simulink model "p03_PID_ZN_SSA_ISSA"  (R2016a)
settings: Solver=VariableStepAuto  StartTime=0.0  StopTime=100  RelTol=1e-3
libraries: simulink x5, dspsrcs4 x1
settings Model: Creator=Administrator  LastModifiedBy=Administrator

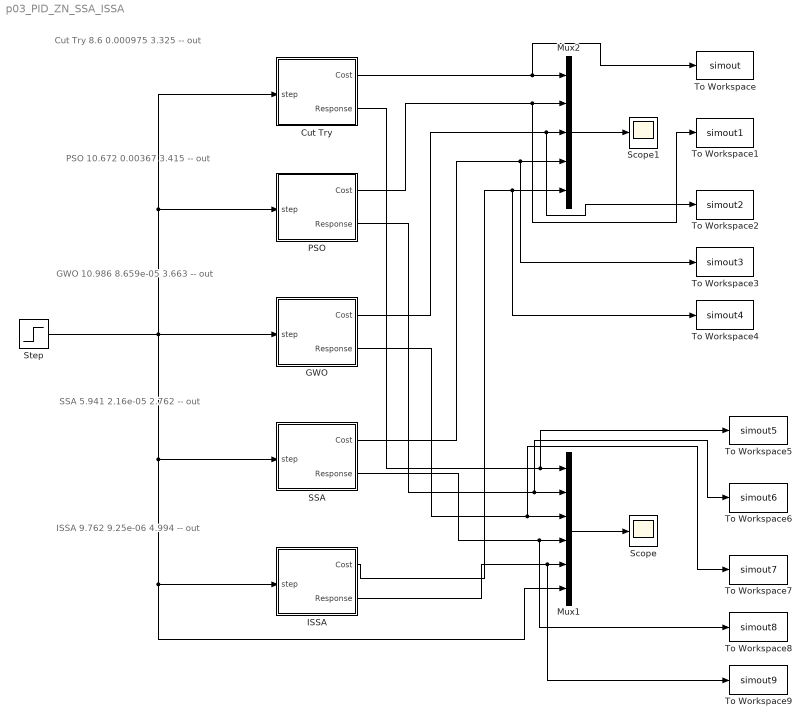
== system p03_PID_ZN_SSA_ISSA ==
  note: ISSA 9.762 9.25e-06 4.994 -- out
  note: SSA 5.941 2.16e-05 2.762 -- out
  note: Cut Try 8.6 0.000975 3.325 -- out
  note: GWO 10.986 8.659e-05 3.663 -- out
  note: PSO 10.672 0.00367 3.415 -- out
  Cut Try : Subsystem
  GWO : Subsystem
  ISSA : Subsystem
  Mux1 : Mux  Inputs=6
  Mux2 : Mux  Inputs=5
  PSO : Subsystem
  SSA : Subsystem
  Scope : Scope
  Scope1 : Scope
  Step : Step  Time=10  SampleTime=0
  To Workspace : ToWorkspace  VariableName=simout  SaveFormat=Timeseries  SampleTime=-1
  To Workspace1 : ToWorkspace  VariableName=simout1  SaveFormat=Timeseries  SampleTime=-1
  To Workspace2 : ToWorkspace  VariableName=simout2  SaveFormat=Timeseries  SampleTime=-1
  To Workspace3 : ToWorkspace  VariableName=simout3  SaveFormat=Timeseries  SampleTime=-1
  To Workspace4 : ToWorkspace  VariableName=simout4  SaveFormat=Timeseries  SampleTime=-1
  To Workspace5 : ToWorkspace  VariableName=simout5  SaveFormat=Timeseries  SampleTime=-1
  To Workspace6 : ToWorkspace  VariableName=simout6  SaveFormat=Timeseries  SampleTime=-1
  To Workspace7 : ToWorkspace  VariableName=simout7  SaveFormat=Timeseries  SampleTime=-1
  To Workspace8 : ToWorkspace  VariableName=simout8  SaveFormat=Timeseries  SampleTime=-1
  To Workspace9 : ToWorkspace  VariableName=simout9  SaveFormat=Timeseries  SampleTime=-1
  wires:
  Mux1/1 -> Scope/1
  Mux2/1 -> Scope1/1
  Step/1 -> GWO/1(step), PSO/1(step), Cut Try/1(step), Mux1/6, ISSA/1(step), SSA/1(step)
  Cut Try/1(Cost) -> To Workspace/1, Mux2/1
  Cut Try/2(Response) -> To Workspace5/1, Mux1/1
  PSO/1(Cost) -> To Workspace1/1, Mux2/2
  PSO/2(Response) -> To Workspace6/1, Mux1/2
  GWO/1(Cost) -> To Workspace2/1, Mux2/3
  GWO/2(Response) -> To Workspace7/1, Mux1/3
  SSA/1(Cost) -> To Workspace3/1, Mux2/4
  SSA/2(Response) -> To Workspace8/1, Mux1/4
  ISSA/1(Cost) -> To Workspace4/1, Mux2/5
  ISSA/2(Response) -> To Workspace9/1, Mux1/5

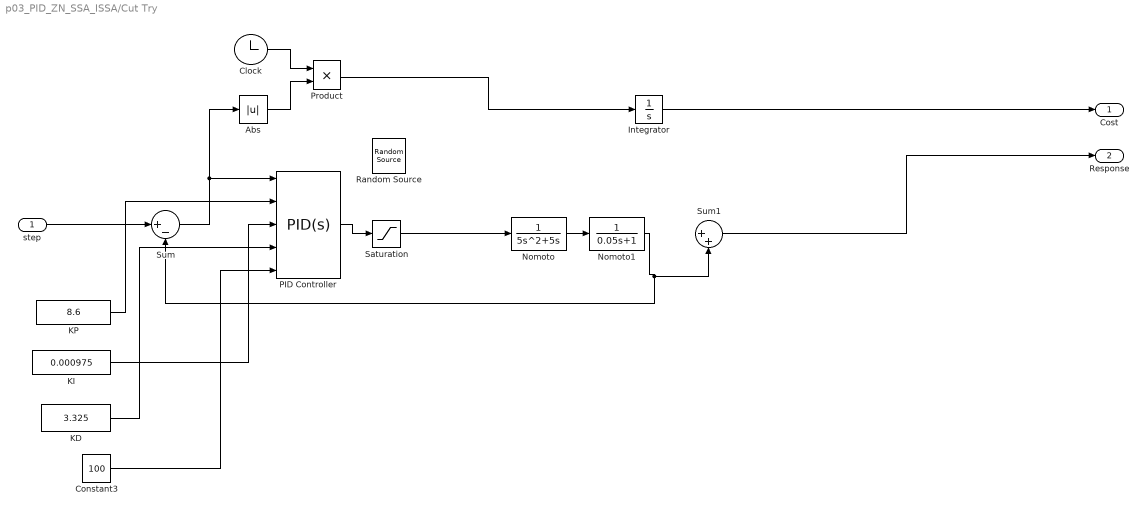
== system p03_PID_ZN_SSA_ISSA/Cut Try ==
  step : Inport
  Abs : Abs
  Clock : Clock
  Constant3 : Constant  Value=100
  Integrator : Integrator
  KD : Constant  Value=3.325
  KI : Constant  Value=0.000975
  KP : Constant  Value=8.6
  Nomoto : TransferFcn  Denominator=[5 5 0]
  Nomoto1 : TransferFcn  Denominator=[0.05 1]
  PID Controller : simulink/Continuous/PID Controller  Controller=PID  TimeDomain=Continuous-time  SampleTime=-1  IntegratorMethod=Forward Euler  FilterMethod=Forward Euler  Form=Parallel  UseFilter=on  ControllerParametersSource=external  P=1  I=1  D=0  N=100  InitialConditionSource=internal  InitialConditionForIntegrator=0  InitialConditionForFilter=0  ExternalReset=none  IgnoreLimit=on  ZeroCross=off  LimitOutput=off  UpperSaturationLimit=inf  LowerSaturationLimit=-inf  LinearizeAsGain=on  AntiWindupMode=none  Kb=1  TrackingMode=off  Kt=1  PParamMin=[]  PParamMax=[]  IParamMin=[]  IParamMax=[]  DParamMin=[]  DParamMax=[]  NParamMin=[]  NParamMax=[]  KbParamMin=[]  KbParamMax=[]  KtParamMin=[]  KtParamMax=[]  POutMin=[]  POutMax=[]  IOutMin=[]  IOutMax=[]  DOutMin=[]  DOutMax=[]  NOutMin=[]  NOutMax=[]  KbOutMin=[]  KbOutMax=[]  KtOutMin=[]  KtOutMax=[]  IntegratorOutMin=[]  IntegratorOutMax=[]  FilterOutMin=[]  FilterOutMax=[]  SumOutMin=[]  SumOutMax=[]  SumI1OutMin=[]  SumI1OutMax=[]  SumI2OutMin=[]  SumI2OutMax=[]  SumI3OutMin=[]  SumI3OutMax=[]  SumDOutMin=[]  SumDOutMax=[]  SaturationOutMin=[]  SaturationOutMax=[]  IntegratorContinuousStateAttributes=''  IntegratorStateMustResolveToSignalObject=off  IntegratorRTWStateStorageClass=Auto  FilterContinuousStateAttributes=''  FilterStateMustResolveToSignalObject=off  FilterRTWStateStorageClass=Auto  DifferentiatorICPrevScaledInput=0  DifferentiatorOutMin=[]  DifferentiatorOutMax=[]
  Product : Product
  Random Source : dspsrcs4/Random Source  SrcType=Gaussian  NormMethod=Ziggurat  CltLength=12  MinVal=0  MaxVal=1  MeanVal=0  VarVal=0.0001  RepMode=Not repeatable  rawSeed=1  IsInherit=off  SampMode=Discrete  SampTime=1  SampFrame=1  DataType=Double  OutComplex=Real  OutputFrames=off
  Saturation : Saturate  UpperLimit=2  LowerLimit=-2
  Sum : Sum  Inputs=|+-
  Sum1 : Sum  Inputs=|++
  Cost : Outport
  Response : Outport  Port=2
  wires:
  Nomoto/1 -> Nomoto1/1
  Clock/1 -> Product/1
  Sum/1 -> Abs/1, PID Controller/1
  Product/1 -> Integrator/1
  Abs/1 -> Product/2
  step/1 -> Sum/1
  Integrator/1 -> Cost/1
  PID Controller/1 -> Saturation/1
  Constant3/1 -> PID Controller/5
  KD/1 -> PID Controller/4
  KI/1 -> PID Controller/3
  KP/1 -> PID Controller/2
  Nomoto1/1 -> Sum1/2, Sum/2
  Saturation/1 -> Nomoto/1
  Sum1/1 -> Response/1

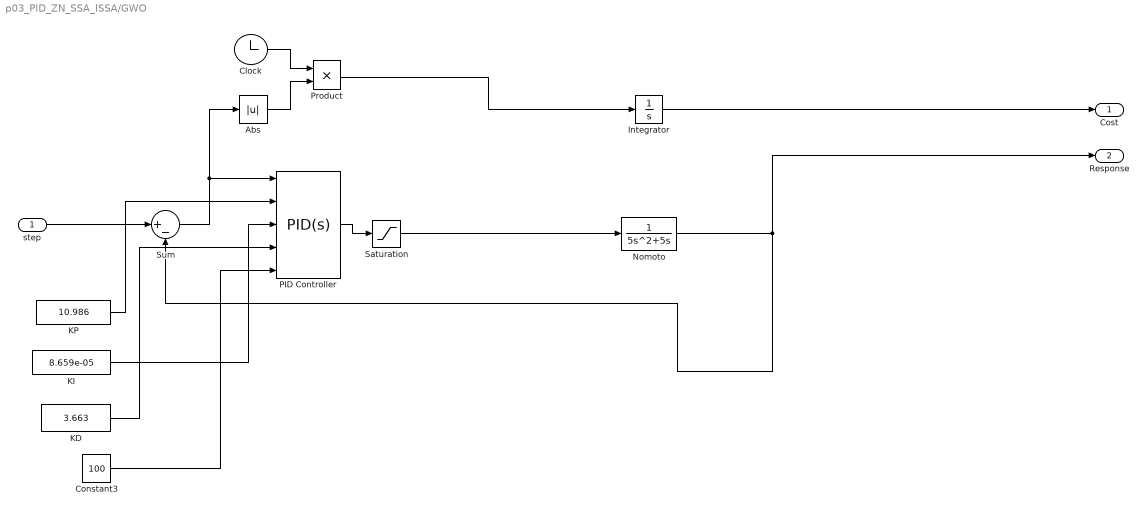
== system p03_PID_ZN_SSA_ISSA/GWO ==
  step : Inport
  Abs : Abs
  Clock : Clock
  Constant3 : Constant  Value=100
  Integrator : Integrator
  KD : Constant  Value=3.663
  KI : Constant  Value=8.659e-05
  KP : Constant  Value=10.986
  Nomoto : TransferFcn  Denominator=[5 5 0]
  PID Controller : simulink/Continuous/PID Controller  Controller=PID  TimeDomain=Continuous-time  SampleTime=-1  IntegratorMethod=Forward Euler  FilterMethod=Forward Euler  Form=Parallel  UseFilter=on  ControllerParametersSource=external  P=1  I=1  D=0  N=100  InitialConditionSource=internal  InitialConditionForIntegrator=0  InitialConditionForFilter=0  ExternalReset=none  ZeroCross=off  LimitOutput=off  UpperSaturationLimit=inf  LowerSaturationLimit=-inf  LinearizeAsGain=on  AntiWindupMode=none  Kb=1  TrackingMode=off  Kt=1  PParamMin=[]  PParamMax=[]  IParamMin=[]  IParamMax=[]  DParamMin=[]  DParamMax=[]  NParamMin=[]  NParamMax=[]  KbParamMin=[]  KbParamMax=[]  KtParamMin=[]  KtParamMax=[]  POutMin=[]  POutMax=[]  IOutMin=[]  IOutMax=[]  DOutMin=[]  DOutMax=[]  NOutMin=[]  NOutMax=[]  KbOutMin=[]  KbOutMax=[]  KtOutMin=[]  KtOutMax=[]  IntegratorOutMin=[]  IntegratorOutMax=[]  FilterOutMin=[]  FilterOutMax=[]  SumOutMin=[]  SumOutMax=[]  SumI1OutMin=[]  SumI1OutMax=[]  SumI2OutMin=[]  SumI2OutMax=[]  SumI3OutMin=[]  SumI3OutMax=[]  SumDOutMin=[]  SumDOutMax=[]  SaturationOutMin=[]  SaturationOutMax=[]  IntegratorContinuousStateAttributes=''  IntegratorStateMustResolveToSignalObject=off  IntegratorRTWStateStorageClass=Auto  FilterContinuousStateAttributes=''  FilterStateMustResolveToSignalObject=off  FilterRTWStateStorageClass=Auto  DifferentiatorICPrevScaledInput=0  DifferentiatorOutMin=[]  DifferentiatorOutMax=[]
  Product : Product
  Saturation : Saturate  UpperLimit=2  LowerLimit=-2
  Sum : Sum  Inputs=|+-
  Cost : Outport
  Response : Outport  Port=2
  wires:
  Nomoto/1 -> Response/1, Sum/2
  Clock/1 -> Product/1
  Sum/1 -> Abs/1, PID Controller/1
  Product/1 -> Integrator/1
  Saturation/1 -> Nomoto/1
  Abs/1 -> Product/2
  step/1 -> Sum/1
  Integrator/1 -> Cost/1
  PID Controller/1 -> Saturation/1
  Constant3/1 -> PID Controller/5
  KD/1 -> PID Controller/4
  KI/1 -> PID Controller/3
  KP/1 -> PID Controller/2

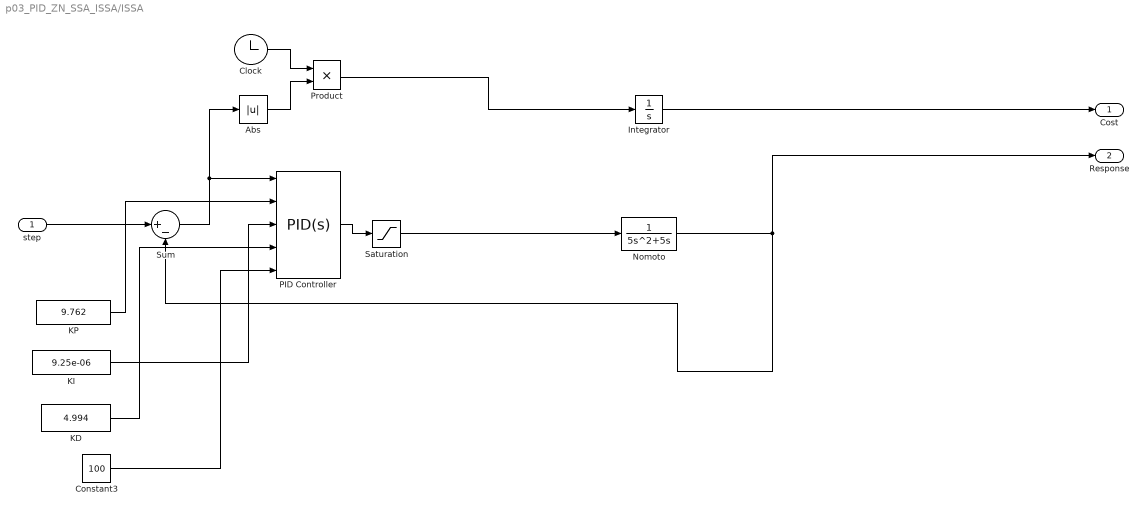
== system p03_PID_ZN_SSA_ISSA/ISSA ==
  step : Inport
  Abs : Abs
  Clock : Clock
  Constant3 : Constant  Value=100
  Integrator : Integrator
  KD : Constant  Value=4.994
  KI : Constant  Value=9.25e-06
  KP : Constant  Value=9.762
  Nomoto : TransferFcn  Denominator=[5 5 0]
  PID Controller : simulink/Continuous/PID Controller  Controller=PID  TimeDomain=Continuous-time  SampleTime=-1  IntegratorMethod=Forward Euler  FilterMethod=Forward Euler  Form=Parallel  UseFilter=on  ControllerParametersSource=external  P=1  I=1  D=0  N=100  InitialConditionSource=internal  InitialConditionForIntegrator=0  InitialConditionForFilter=0  ExternalReset=none  ZeroCross=off  LimitOutput=off  UpperSaturationLimit=inf  LowerSaturationLimit=-inf  LinearizeAsGain=on  AntiWindupMode=none  Kb=1  TrackingMode=off  Kt=1  PParamMin=[]  PParamMax=[]  IParamMin=[]  IParamMax=[]  DParamMin=[]  DParamMax=[]  NParamMin=[]  NParamMax=[]  KbParamMin=[]  KbParamMax=[]  KtParamMin=[]  KtParamMax=[]  POutMin=[]  POutMax=[]  IOutMin=[]  IOutMax=[]  DOutMin=[]  DOutMax=[]  NOutMin=[]  NOutMax=[]  KbOutMin=[]  KbOutMax=[]  KtOutMin=[]  KtOutMax=[]  IntegratorOutMin=[]  IntegratorOutMax=[]  FilterOutMin=[]  FilterOutMax=[]  SumOutMin=[]  SumOutMax=[]  SumI1OutMin=[]  SumI1OutMax=[]  SumI2OutMin=[]  SumI2OutMax=[]  SumI3OutMin=[]  SumI3OutMax=[]  SumDOutMin=[]  SumDOutMax=[]  SaturationOutMin=[]  SaturationOutMax=[]  IntegratorContinuousStateAttributes=''  IntegratorStateMustResolveToSignalObject=off  IntegratorRTWStateStorageClass=Auto  FilterContinuousStateAttributes=''  FilterStateMustResolveToSignalObject=off  FilterRTWStateStorageClass=Auto  DifferentiatorICPrevScaledInput=0  DifferentiatorOutMin=[]  DifferentiatorOutMax=[]
  Product : Product
  Saturation : Saturate  UpperLimit=2  LowerLimit=-2
  Sum : Sum  Inputs=|+-
  Cost : Outport
  Response : Outport  Port=2
  wires:
  Nomoto/1 -> Response/1, Sum/2
  Clock/1 -> Product/1
  Sum/1 -> Abs/1, PID Controller/1
  Product/1 -> Integrator/1
  Saturation/1 -> Nomoto/1
  Abs/1 -> Product/2
  step/1 -> Sum/1
  Integrator/1 -> Cost/1
  PID Controller/1 -> Saturation/1
  Constant3/1 -> PID Controller/5
  KD/1 -> PID Controller/4
  KI/1 -> PID Controller/3
  KP/1 -> PID Controller/2

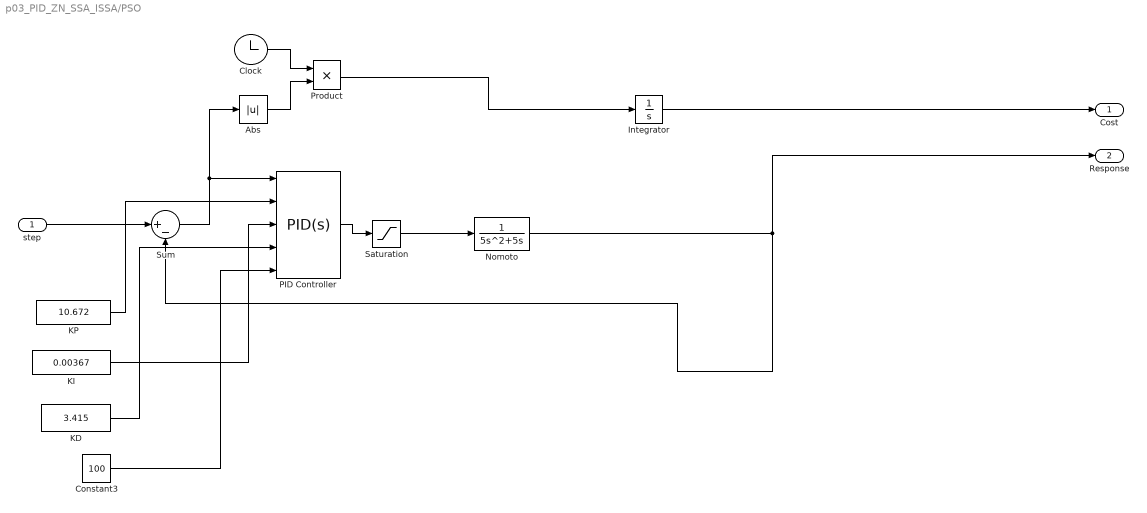
== system p03_PID_ZN_SSA_ISSA/PSO ==
  step : Inport
  Abs : Abs
  Clock : Clock
  Constant3 : Constant  Value=100
  Integrator : Integrator
  KD : Constant  Value=3.415
  KI : Constant  Value=0.00367
  KP : Constant  Value=10.672
  Nomoto : TransferFcn  Denominator=[5 5 0]
  PID Controller : simulink/Continuous/PID Controller  Controller=PID  TimeDomain=Continuous-time  SampleTime=-1  IntegratorMethod=Forward Euler  FilterMethod=Forward Euler  Form=Parallel  UseFilter=on  ControllerParametersSource=external  P=1  I=1  D=0  N=100  InitialConditionSource=internal  InitialConditionForIntegrator=0  InitialConditionForFilter=0  ExternalReset=none  ZeroCross=off  LimitOutput=off  UpperSaturationLimit=inf  LowerSaturationLimit=-inf  LinearizeAsGain=on  AntiWindupMode=none  Kb=1  TrackingMode=off  Kt=1  PParamMin=[]  PParamMax=[]  IParamMin=[]  IParamMax=[]  DParamMin=[]  DParamMax=[]  NParamMin=[]  NParamMax=[]  KbParamMin=[]  KbParamMax=[]  KtParamMin=[]  KtParamMax=[]  POutMin=[]  POutMax=[]  IOutMin=[]  IOutMax=[]  DOutMin=[]  DOutMax=[]  NOutMin=[]  NOutMax=[]  KbOutMin=[]  KbOutMax=[]  KtOutMin=[]  KtOutMax=[]  IntegratorOutMin=[]  IntegratorOutMax=[]  FilterOutMin=[]  FilterOutMax=[]  SumOutMin=[]  SumOutMax=[]  SumI1OutMin=[]  SumI1OutMax=[]  SumI2OutMin=[]  SumI2OutMax=[]  SumI3OutMin=[]  SumI3OutMax=[]  SumDOutMin=[]  SumDOutMax=[]  SaturationOutMin=[]  SaturationOutMax=[]  IntegratorContinuousStateAttributes=''  IntegratorStateMustResolveToSignalObject=off  IntegratorRTWStateStorageClass=Auto  FilterContinuousStateAttributes=''  FilterStateMustResolveToSignalObject=off  FilterRTWStateStorageClass=Auto  DifferentiatorICPrevScaledInput=0  DifferentiatorOutMin=[]  DifferentiatorOutMax=[]
  Product : Product
  Saturation : Saturate  UpperLimit=2  LowerLimit=-2
  Sum : Sum  Inputs=|+-
  Cost : Outport
  Response : Outport  Port=2
  wires:
  Nomoto/1 -> Response/1, Sum/2
  Clock/1 -> Product/1
  Sum/1 -> Abs/1, PID Controller/1
  Product/1 -> Integrator/1
  Saturation/1 -> Nomoto/1
  Abs/1 -> Product/2
  step/1 -> Sum/1
  Integrator/1 -> Cost/1
  PID Controller/1 -> Saturation/1
  Constant3/1 -> PID Controller/5
  KD/1 -> PID Controller/4
  KI/1 -> PID Controller/3
  KP/1 -> PID Controller/2

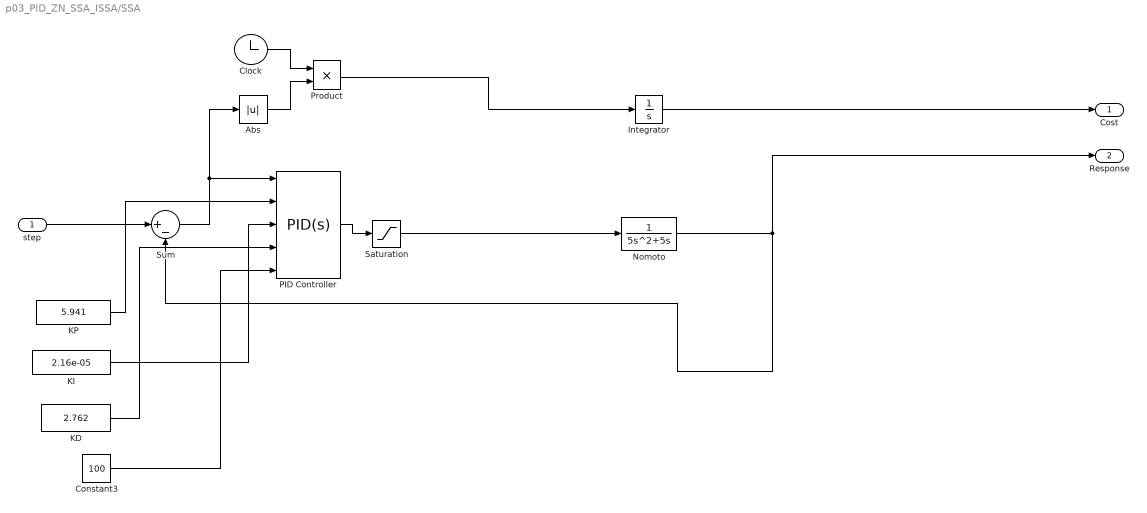
== system p03_PID_ZN_SSA_ISSA/SSA ==
  step : Inport
  Abs : Abs
  Clock : Clock
  Constant3 : Constant  Value=100
  Integrator : Integrator
  KD : Constant  Value=2.762
  KI : Constant  Value=2.16e-05
  KP : Constant  Value=5.941
  Nomoto : TransferFcn  Denominator=[5 5 0]
  PID Controller : simulink/Continuous/PID Controller  Controller=PID  TimeDomain=Continuous-time  SampleTime=-1  IntegratorMethod=Forward Euler  FilterMethod=Forward Euler  Form=Parallel  UseFilter=on  ControllerParametersSource=external  P=1  I=1  D=0  N=100  InitialConditionSource=internal  InitialConditionForIntegrator=0  InitialConditionForFilter=0  ExternalReset=none  ZeroCross=off  LimitOutput=off  UpperSaturationLimit=inf  LowerSaturationLimit=-inf  LinearizeAsGain=on  AntiWindupMode=none  Kb=1  TrackingMode=off  Kt=1  PParamMin=[]  PParamMax=[]  IParamMin=[]  IParamMax=[]  DParamMin=[]  DParamMax=[]  NParamMin=[]  NParamMax=[]  KbParamMin=[]  KbParamMax=[]  KtParamMin=[]  KtParamMax=[]  POutMin=[]  POutMax=[]  IOutMin=[]  IOutMax=[]  DOutMin=[]  DOutMax=[]  NOutMin=[]  NOutMax=[]  KbOutMin=[]  KbOutMax=[]  KtOutMin=[]  KtOutMax=[]  IntegratorOutMin=[]  IntegratorOutMax=[]  FilterOutMin=[]  FilterOutMax=[]  SumOutMin=[]  SumOutMax=[]  SumI1OutMin=[]  SumI1OutMax=[]  SumI2OutMin=[]  SumI2OutMax=[]  SumI3OutMin=[]  SumI3OutMax=[]  SumDOutMin=[]  SumDOutMax=[]  SaturationOutMin=[]  SaturationOutMax=[]  IntegratorContinuousStateAttributes=''  IntegratorStateMustResolveToSignalObject=off  IntegratorRTWStateStorageClass=Auto  FilterContinuousStateAttributes=''  FilterStateMustResolveToSignalObject=off  FilterRTWStateStorageClass=Auto  DifferentiatorICPrevScaledInput=0  DifferentiatorOutMin=[]  DifferentiatorOutMax=[]
  Product : Product
  Saturation : Saturate  UpperLimit=2  LowerLimit=-2
  Sum : Sum  Inputs=|+-
  Cost : Outport
  Response : Outport  Port=2
  wires:
  Nomoto/1 -> Response/1, Sum/2
  Clock/1 -> Product/1
  Sum/1 -> Abs/1, PID Controller/1
  Product/1 -> Integrator/1
  Saturation/1 -> Nomoto/1
  Abs/1 -> Product/2
  step/1 -> Sum/1
  Integrator/1 -> Cost/1
  PID Controller/1 -> Saturation/1
  Constant3/1 -> PID Controller/5
  KD/1 -> PID Controller/4
  KI/1 -> PID Controller/3
  KP/1 -> PID Controller/2
